simulink model "SOC_EKF"  (R2023b)
settings: Solver=FixedStepAuto  StartTime=0.0  StopTime=3600  RelTol=1e-3
undefined symbols (not defined in the file or in its folder): Ion, Lithium
libraries: autolibrcnetworksystem x4, spsBatteryLib x1, spsSeriesRLCBranchLib x1, spspowerguiLib x1
settings Model: Creator=LEGION  LastModifiedBy=LEGION
settings SolverCC: AlgebraicLoopSolver=TrustRegion
settings DebuggingCC: UnconnectedInputMsg=warning  UnconnectedOutputMsg=warning  UnconnectedLineMsg=warning
settings ModelReferenceCC: EnableRefExpFcnMdlSchedulingChecks=on

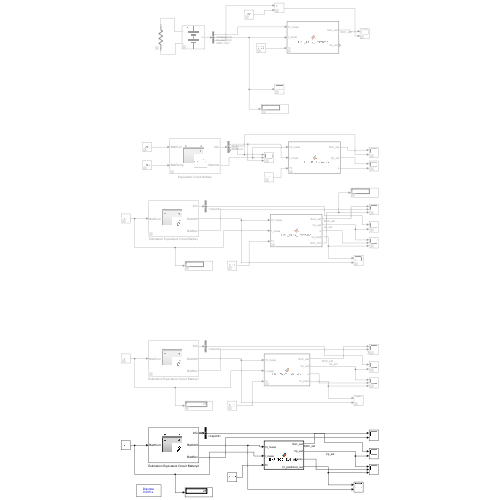
[thumbnail: Simulink's stored preview of the top-level diagram]
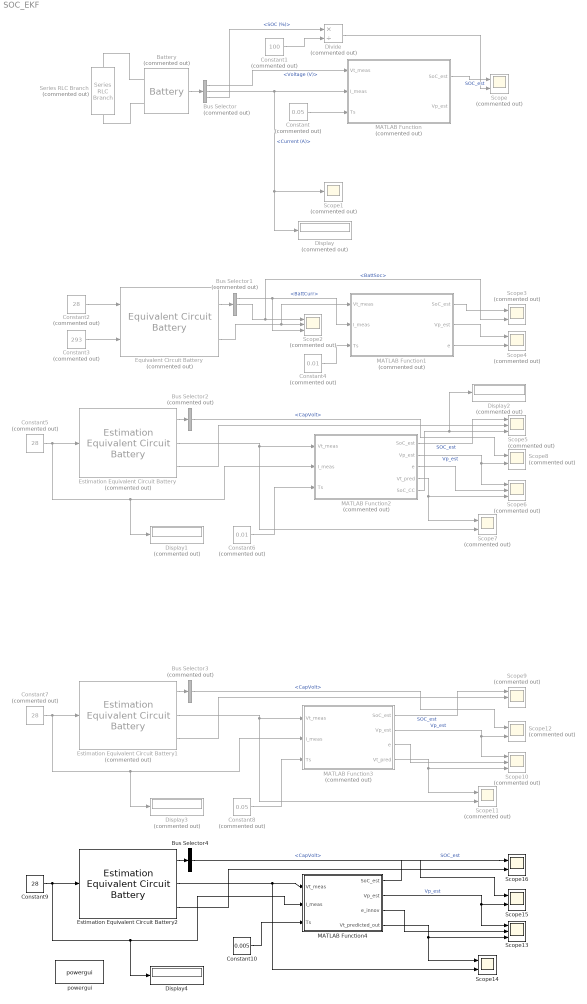
== system SOC_EKF ==
  Battery : spsBatteryLib/Battery  Commented=on  BatType=Lithium-Ion  ShowTempParam=off  ThermalPreset=no  ShowAgeParam=off  NomV=3.7  NomQ=2.3  SOC=85  Batt_Tr=30  PresetModel=on  MaxQ=2.3  MinV=2.775  FullV=4.3068  Dis_rate=1  R=0.016087  Normal_OP=2.08  expZone="[3.9974       0.113]"  current=[6.5 13 32.5]  Units=Time  Tci=20  NomT=20  T2=-30  MaxQ2=4.8  FullV2=7.1  Normal_OP2=5.655  expZone2="[6.58           1]"  Rca=0.6  ti=2000  Dp=0  Neq0=0  Tsim=1e6  Ta1=25  Qeol=5.4*0.9  Reol=0.013333*1.2  Char_age=[2.3478, 3]  Dis_age=[2.3478, 10]  N1=1500  N2=10500  N3=1000  N4=1400  Ta2=45  N5=950
      settings: LibrarySourceBlock=electricdrivelib/Extra Sources/Battery
  Bus Selector : BusSelector  Commented=on  OutputSignals=Voltage (V),Current (A),SOC (%)
  Bus Selector1 : BusSelector  Commented=on  OutputSignals=BattCurr,BattSoc,BattVolt
  Bus Selector2 : BusSelector  Commented=on  OutputSignals=CapVolt
  Bus Selector3 : BusSelector  Commented=on  OutputSignals=CapVolt
  Bus Selector4 : BusSelector  OutputSignals=CapVolt
  Constant : Constant  Commented=on  Value=0.05
  Constant1 : Constant  Commented=on  Value=100
  Constant10 : Constant  Value=0.005
  Constant2 : Constant  Commented=on  Value=28
  Constant3 : Constant  Commented=on  Value=293
  Constant4 : Constant  Commented=on  Value=0.01
  Constant5 : Constant  Commented=on  Value=28
  Constant6 : Constant  Commented=on  Value=0.01
  Constant7 : Constant  Commented=on  Value=28
  Constant8 : Constant  Commented=on  Value=0.05
  Constant9 : Constant  Value=28
  Display{,1..3} (4 alike) : Display  Commented=on
  Display4 : Display
  Divide : Product  Commented=on  Inputs=*/
  Equivalent Circuit Battery : autolibrcnetworksystem/Equivalent Circuit Battery  Commented=on  CapacityCtrl=Parameter  OutputVlt=Unfiltered  NumRC=1  Em=|  R0=|  SOC_BP=|  Temperature_BP=[293.15 313.15]  BattCap=[28 28]  BattCapInit=28  InitialCapVoltage=0  Tc=1/1000  Vinit=4.193  R1=|  C1=|  R2=|  C2=|  R3=|  C3=|  R4=|  C4=|  R5=|  C5=|  Vu=Inf  Vl=-Inf  RefBlkName='autolibrcnetworksystem/Equivalent Circuit Battery'
      Em=|
      | [3.5042 3.5136;
      | 3.5573 3.5646;
      | 3.6009 3.6153;
      | 3.6393 3.6565;
      | 3.6742 3.6889;
      | 3.7121 3.7214;
      | 3.7937 3.8078;
      | 3.8753 3.8945;
      | 3.97 3.9859;
      | 4.0764 4.0821;
      | 4.1924 4.193]
      R0=|
      | [0.011448 0.0090006;
      | 0.011038 0.0089655;
      | 0.011281 0.0091261;
      | 0.011236 0.0091099;
      | 0.010959 0.008957;
      | 0.010714 0.0087969;
      | 0.010698 0.0089126;
      | 0.010712 0.0090517;
      | 0.010917 0.0090444;
      | 0.011304 0.0088992;
      | 0.011603 0.0089015
      | ]
      SOC_BP=|
      | [0
      | 0.1
      | 0.2
      | 0.3
      | 0.4
      | 0.5
      | 0.6
      | 0.7
      | 0.8
      | 0.9
      | 1]
      R1=|
      | [0.010342 0.0012244;
      | 0.0067316 0.0011396;
      | 0.0051156 0.0012661;
      | 0.0043447 0.0012265;
      | 0.0038826 0.0011163;
      | 0.0034226 0.0009968;
      | 0.003346 0.0011458;
      | 0.0033222 0.001345;
      | 0.0033201 0.0013091;
      | 0.0032886 0.0010986;
      | 0.0028114 0.0010309]
      C1=|
      | [2287.7 11897;
      | 6122 24515;
      | 18460 42098;
      | 20975 44453;
      | 15254 33098;
      | 10440 24492;
      | 13903 32975;
      | 16694 40007;
      | 15784 35937;
      | 12165 26430;
      | 9118 24795]
      R2=|
      | [0.010342 0.0012244;
      | 0.0067316 0.0011396;
      | 0.0051156 0.0012661;
      | 0.0043447 0.0012265;
      | 0.0038826 0.0011163;
      | 0.0034226 0.0009968;
      | 0.003346 0.0011458;
      | 0.0033222 0.001345;
      | 0.0033201 0.0013091;
      | 0.0032886 0.0010986;
      | 0.0028114 0.0010309]
      C2=|
      | [2287.7 11897;
      | 6122 24515;
      | 18460 42098;
      | 20975 44453;
      | 15254 33098;
      | 10440 24492;
      | 13903 32975;
      | 16694 40007;
      | 15784 35937;
      | 12165 26430;
      | 9118 24795]
      R3=|
      | [0.010342 0.0012244;
      | 0.0067316 0.0011396;
      | 0.0051156 0.0012661;
      | 0.0043447 0.0012265;
      | 0.0038826 0.0011163;
      | 0.0034226 0.0009968;
      | 0.003346 0.0011458;
      | 0.0033222 0.001345;
      | 0.0033201 0.0013091;
      | 0.0032886 0.0010986;
      | 0.0028114 0.0010309]
      C3=|
      | [2287.7 11897;
      | 6122 24515;
      | 18460 42098;
      | 20975 44453;
      | 15254 33098;
      | 10440 24492;
      | 13903 32975;
      | 16694 40007;
      | 15784 35937;
      | 12165 26430;
      | 9118 24795]
      R4=|
      | [0.010342 0.0012244;
      | 0.0067316 0.0011396;
      | 0.0051156 0.0012661;
      | 0.0043447 0.0012265;
      | 0.0038826 0.0011163;
      | 0.0034226 0.0009968;
      | 0.003346 0.0011458;
      | 0.0033222 0.001345;
      | 0.0033201 0.0013091;
      | 0.0032886 0.0010986;
      | 0.0028114 0.0010309]
      C4=|
      | [2287.7 11897;
      | 6122 24515;
      | 18460 42098;
      | 20975 44453;
      | 15254 33098;
      | 10440 24492;
      | 13903 32975;
      | 16694 40007;
      | 15784 35937;
      | 12165 26430;
      | 9118 24795]
      R5=|
      | [0.010342 0.0012244;
      | 0.0067316 0.0011396;
      | 0.0051156 0.0012661;
      | 0.0043447 0.0012265;
      | 0.0038826 0.0011163;
      | 0.0034226 0.0009968;
      | 0.003346 0.0011458;
      | 0.0033222 0.001345;
      | 0.0033201 0.0013091;
      | 0.0032886 0.0010986;
      | 0.0028114 0.0010309]
      C5=|
      | [2287.7 11897;
      | 6122 24515;
      | 18460 42098;
      | 20975 44453;
      | 15254 33098;
      | 10440 24492;
      | 13903 32975;
      | 16694 40007;
      | 15784 35937;
      | 12165 26430;
      | 9118 24795]
  Estimation Equivalent Circuit Battery : autolibrcnetworksystem/Estimation Equivalent Circuit Battery  Commented=on  NumRC=1  Em=[2.775 3 3.7 3.8 4 4.3068]  R0=[0.01 0.01 0.01 0.01 0.01 0.01]  SOC_BP=[0 .2 .4 .6 .8 1]  BattCap=28  BattCapInit=28  InitialCapVoltage=0  R1=[0.005 0.005 0.005 0.005 0.005 0.005]  C1=[10000 10000 10000 10000 10000 10000]  R2=[0.005 0.005 0.005 0.005 0.005 0.005]  C2=[10000 10000 10000 10000 10000 10000]  R3=[0.005 0.005 0.005 0.005 0.005 0.005]  C3=[10000 10000 10000 10000 10000 10000]  R4=[0.005 0.005 0.005 0.005 0.005 0.005]  C4=[10000 10000 10000 10000 10000 10000]  R5=[0.005 0.005 0.005 0.005 0.005 0.005]  C5=[10000 10000 10000 10000 10000 10000]  Vu=Inf  Vl=-Inf
  Estimation Equivalent Circuit Battery1 : autolibrcnetworksystem/Estimation Equivalent Circuit Battery  Commented=on  NumRC=1  Em=[2.775 3 3.7 3.8 4 4.3068]  R0=[0.01 0.01 0.01 0.01 0.01 0.01]  SOC_BP=[0 .2 .4 .6 .8 1]  BattCap=28  BattCapInit=28  InitialCapVoltage=0  R1=[0.005 0.005 0.005 0.005 0.005 0.005]  C1=[10000 10000 10000 10000 10000 10000]  R2=[0.005 0.005 0.005 0.005 0.005 0.005]  C2=[10000 10000 10000 10000 10000 10000]  R3=[0.005 0.005 0.005 0.005 0.005 0.005]  C3=[10000 10000 10000 10000 10000 10000]  R4=[0.005 0.005 0.005 0.005 0.005 0.005]  C4=[10000 10000 10000 10000 10000 10000]  R5=[0.005 0.005 0.005 0.005 0.005 0.005]  C5=[10000 10000 10000 10000 10000 10000]  Vu=Inf  Vl=-Inf
  Estimation Equivalent Circuit Battery2 : autolibrcnetworksystem/Estimation Equivalent Circuit Battery  NumRC=1  Em=[2.775 3 3.7 3.8 4 4.3068]  R0=[0.01 0.01 0.01 0.01 0.01 0.01]  SOC_BP=[0 .2 .4 .6 .8 1]  BattCap=28  BattCapInit=28  InitialCapVoltage=0  R1=[0.005 0.005 0.005 0.005 0.005 0.005]  C1=[10000 10000 10000 10000 10000 10000]  R2=[0.005 0.005 0.005 0.005 0.005 0.005]  C2=[10000 10000 10000 10000 10000 10000]  R3=[0.005 0.005 0.005 0.005 0.005 0.005]  C3=[10000 10000 10000 10000 10000 10000]  R4=[0.005 0.005 0.005 0.005 0.005 0.005]  C4=[10000 10000 10000 10000 10000 10000]  R5=[0.005 0.005 0.005 0.005 0.005 0.005]  C5=[10000 10000 10000 10000 10000 10000]  Vu=Inf  Vl=-Inf
  MATLAB Function : MATLAB Function  Commented=on  TreatAsAtomicUnit=on
  MATLAB Function1 : MATLAB Function  Commented=on  TreatAsAtomicUnit=on
  MATLAB Function2 : MATLAB Function  Commented=on  TreatAsAtomicUnit=on
  MATLAB Function3 : MATLAB Function  Commented=on  TreatAsAtomicUnit=on
  MATLAB Function4 : MATLAB Function  TreatAsAtomicUnit=on
  Scope{,3..4,7..8,11..12} (7 alike) : Scope  Commented=on  NumInputPorts=2
  Scope1 : Scope  Commented=on
  Scope{2,5..6,9..10} (5 alike) : Scope  Commented=on  NumInputPorts=3
  Scope13 : Scope  NumInputPorts=3
  Scope14 : Scope  NumInputPorts=2
  Scope15 : Scope  NumInputPorts=2
  Scope16 : Scope  NumInputPorts=2
  Series RLC Branch : spsSeriesRLCBranchLib/Series RLC Branch  Commented=on  LConnTagsString=__new0  RConnTagsString=__new0  BranchType=R  Resistance=1  Inductance=1e-3  SetiL0=off  InitialCurrent=0  Capacitance=1e-6  Setx0=off  InitialVoltage=0  Measurements=None
  powergui : spspowerguiLib/powergui  Priority=1  SimulationMode=Discrete  SampleTime=0.005  frequency=60  Iterations=50  frequencyindice=0  Pbase=100e6  ErrMax=1e-4  UnitsV=kV  UnitsW=MW  buscounter=0  FunctionMessages=off  echomessages=off  EnableUseOfTLC=off  CurrentSourceSwitches=off  DisableSnubberDevices=off  DisableRonSwitches=off  DisableVfSwitches=off  DisplayEquations=off  AutomaticDiscreteSolvers=off  SolverType=Tustin/Backward Euler (TBE)  Interpol=off  ExternalGateDelay=off  methode=off  Ts=100  x0status=blocks  SPID=on  SwTol=0  HookPort=off  NonlinearTolerance=1e-4  nMaxIteration=100  ContinueOnMaxIteration=off  RestoreLinks=warning  ResistiveCurrentMeasurement=off  Frange=[0:2:500]  Ylog=off  Xlog=on  ShowGrid=off  save=off  variable=ZData  structure=0  ZoomFFT=off  StartTime=0.0  cycles=1  DisplayStyle=1  fundamental=60  FreqAxis=off  MaxFrequency=1000  frequencyindicesteady=1  RmsSteady=1  display=off
  wires:
  Battery/1 -> Bus Selector/1
  Bus Selector/1 -> MATLAB Function/1(Vt_meas)  "<Voltage (V)>"
  Bus Selector/2 -> Scope1/1, Display/1, MATLAB Function/2(I_meas)  "<Current (A)>"
  Constant/1 -> MATLAB Function/3(Ts)
  MATLAB Function/1(SoC_est) -> Scope/1  "SOC_est"
  Bus Selector/3 -> Divide/1  "<SOC (%)>"
  Divide/1 -> Scope/2
  Constant1/1 -> Divide/2
  Equivalent Circuit Battery/2 -> MATLAB Function1/1(Vt_meas), Scope2/2
  Constant2/1 -> Equivalent Circuit Battery/1
  Constant3/1 -> Equivalent Circuit Battery/2
  Equivalent Circuit Battery/1 -> Bus Selector1/1
  Bus Selector1/2 -> Scope3/2, Scope2/1  "<BattSoc>"
  Bus Selector1/1 -> Scope2/3, MATLAB Function1/2(I_meas)  "<BattCurr>"
  Constant4/1 -> MATLAB Function1/3(Ts)
  MATLAB Function1/1(SoC_est) -> Scope3/1
  MATLAB Function1/2(Vp_est) -> Scope4/1
  MATLAB Function1/3(e) -> Scope4/2
  Estimation Equivalent Circuit Battery/2 -> Scope7/2, MATLAB Function2/1(Vt_meas)
  Constant5/1 -> Display1/1, MATLAB Function2/2(I_meas), Estimation Equivalent Circuit Battery/1
  MATLAB Function2/1(SoC_est) -> Scope5/1  "SOC_est"
  Estimation Equivalent Circuit Battery/3 -> Scope5/2
  MATLAB Function2/2(Vp_est) -> Scope8/2, Scope6/1  "Vp_est"
  MATLAB Function2/3(e) -> Scope6/2
  MATLAB Function2/4(Vt_pred) -> Scope7/1, Scope6/3
  Constant6/1 -> MATLAB Function2/3(Ts)
  MATLAB Function2/5(SoC_CC) -> Display2/1, Scope5/3
  Estimation Equivalent Circuit Battery/1 -> Bus Selector2/1
  Bus Selector2/1 -> Scope8/1  "<CapVolt>"
  Bus Selector3/1 -> Scope12/1  "<CapVolt>"
  MATLAB Function3/4(Vt_pred) -> Scope11/1, Scope10/3
  Estimation Equivalent Circuit Battery1/3 -> Scope9/2
  Constant8/1 -> MATLAB Function3/3(Ts)
  MATLAB Function3/3(e) -> Scope10/2
  MATLAB Function3/2(Vp_est) -> Scope12/2, Scope10/1  "Vp_est"
  Estimation Equivalent Circuit Battery1/1 -> Bus Selector3/1
  Estimation Equivalent Circuit Battery1/2 -> MATLAB Function3/1(Vt_meas), Scope11/2
  MATLAB Function3/1(SoC_est) -> Scope9/1  "SOC_est"
  Constant7/1 -> MATLAB Function3/2(I_meas), Display3/1, Estimation Equivalent Circuit Battery1/1
  Constant9/1 -> MATLAB Function4/2(I_meas), Display4/1, Estimation Equivalent Circuit Battery2/1
  Estimation Equivalent Circuit Battery2/1 -> Bus Selector4/1
  MATLAB Function4/3(e_innov) -> Scope13/2
  MATLAB Function4/1(SoC_est) -> Scope16/1  "SOC_est"
  Estimation Equivalent Circuit Battery2/2 -> Scope14/2, MATLAB Function4/1(Vt_meas)
  MATLAB Function4/2(Vp_est) -> Scope15/2, Scope13/1  "Vp_est"
  MATLAB Function4/4(Vt_predicted_out) -> Scope14/1, Scope13/3
  Estimation Equivalent Circuit Battery2/3 -> Scope16/2
  Bus Selector4/1 -> Scope15/1  "<CapVolt>"
  Constant10/1 -> MATLAB Function4/3(Ts)
  connections:
  Series RLC Branch/LConn1 -- Battery/LConn1
  Series RLC Branch/RConn1 -- Battery/LConn2

== matlab function SOC_EKF/MATLAB Function1 ==
  settings: updateMethod=DISCRETE
  data: Vt_meas input; SoC_est output; I_meas input; Ts input; Vp_est output; e output
function [SoC_est, Vp_est, e] = EKF_SOC_Estimator(Vt_meas, I_meas, Ts)

% ---------------------------- Persistent Variables ----------------------------
persistent x P Q R
persistent SoC_vec Em_chg Em_dis R0_chg R0_dis R1_chg R1_dis C1_table_chg C1_table_dis
persistent BattCapInit initialized

if isempty(initialized)
    initialized = true;

    % 11-point SoC vector (even spacing)
    SoC_vec = linspace(0, 1, 11);

    % Lookup table data
    Em = [3.5042 3.5136;
          3.5573 3.5646;
          3.6009 3.6153;
          3.6393 3.6565;
          3.6742 3.6889;
          3.7121 3.7214;
          3.7937 3.8078;
          3.8753 3.8945;
          3.9700 3.9859;
          4.0764 4.0821;
          4.1924 4.1930];

    R0 = [0.011448 0.0090006;
          0.011038 0.0089655;
          0.011281 0.0091261;
          0.011236 0.0091099;
          0.010959 0.0089570;
          0.010714 0.0087969;
          0.010698 0.0089126;
          0.010712 0.0090517;
          0.010917 0.0090444;
          0.011304 0.0088992;
          0.011603 0.0089015];

    R1 = [0.010342 0.0012244;
          0.0067316 0.0011396;
          0.0051156 0.0012661;
          0.0043447 0.0012265;
          0.0038826 0.0011163;
          0.0034226 0.0009968;
          0.0033460 0.0011458;
          0.0033222 0.0013450;
          0.0033201 0.0013091;
          0.0032886 0.0010986;
          0.0028114 0.0010309];

    C1_table = [2287.7 11897;
                6122   24515;
               18460   42098;
               20975   44453;
               15254   33098;
               10440   24492;
               13903   32975;
               16694   40007;
               15784   35937;
               12165   26430;
                9118   24795];

    % Split into charge/discharge
    Em_dis = Em(:,1); Em_chg = Em(:,2);
    R0_dis = R0(:,1); R0_chg = R0(:,2);
    R1_dis = R1(:,1); R1_chg = R1(:,2);
    C1_table_dis = C1_table(:,1); C1_table_chg = C1_table(:,2);

    % Battery capacity
    BattCapInit = 28;  % [Ah]

    % ---------------- Initial State (Realistic) ----------------
    SoC_init = 1.0;
    Voc_init = Em_dis(end);  % Voc at 100% SoC
    Rt_init  = R0_dis(end);  % Rt at 100% SoC
    Vp_init  = Voc_init - Vt_meas + Rt_init * I_meas;

    x = [SoC_init; Vp_init];

    % Initial covariance
    P = 1e-2 * eye(2);

    % Noise covariance
    Q = diag([1e-4, 1e-3]);
    R = 1e-2;

end

% ---------------------------- Parameter Interpolation ----------------------------
SoC = min(max(x(1), 0), 1);  % Clamp SoC to [0,1]

if I_meas >= 0  % Discharge
    Voc = interp1(SoC_vec, Em_dis, SoC, 'linear', 'extrap');
    Rt  = interp1(SoC_vec, R0_dis, SoC, 'linear', 'extrap');
    Rp  = interp1(SoC_vec, R1_dis, SoC, 'linear', 'extrap');
    Cp  = interp1(SoC_vec, C1_table_dis, SoC, 'linear', 'extrap');
else
    Voc = interp1(SoC_vec, Em_chg, SoC, 'linear', 'extrap');
    Rt  = interp1(SoC_vec, R0_chg, SoC, 'linear', 'extrap');
    Rp  = interp1(SoC_vec, R1_chg, SoC, 'linear', 'extrap');
    Cp  = interp1(SoC_vec, C1_table_chg, SoC, 'linear', 'extrap');
end

Cp = max(Cp, 1e-3);  % Prevent numerical issues

% ---------------------------- Discrete-Time Model ----------------------------
alpha = exp(-Ts / (Rp * Cp));
A = [1, 0;
     0, alpha];
B = [-Ts / (3600 * BattCapInit);
      Rp * (1 - alpha)];

% ---------------------------- EKF PREDICTION ----------------------------
x_pred = A * x + B * I_meas;
P_pred = A * P * A' + Q;

% ---------------------------- Measurement Prediction ----------------------------
Vt_pred = Voc - x_pred(2) + Rt * I_meas;

% ---------------------------- Correction ----------------------------
C_k = [1, -1];
e = Vt_meas - Vt_pred;
S_k = C_k * P_pred * C_k' + R;
K = P_pred * C_k' / S_k;

x = x_pred + K * e;
P = (eye(2) - K * C_k) * P_pred;

% ---------------------------- Output ----------------------------
SoC_est = max(0, min(1, x(1)));
Vp_est  = x(2);
e = Vt_meas - Vt_pred;

end

== matlab function SOC_EKF/MATLAB Function ==
  data: Vt_meas input; SoC_est output; I_meas input; Ts input; Vp_est output
function [SoC_est, Vp_est] = EKF_SOC_Estimator(Vt_meas, I_meas, Ts)

% --- Persistent variables to retain state across time steps ---
persistent x P Q R A B C D Voc0 dVoc C_nom Rp Cp

if isempty(x)
    % Initial state: SoC (0.85) and Vp (0 V)
    x = [0.85; 0];  % [SoC; Vp]

    % Covariance matrix (uncertainty in initial estimate)
    P = 1e-2 * eye(2);

    % Process noise covariance (uncertainty in model)
    Q = diag([1e-6, 1e-4]);

    % Measurement noise covariance (voltage sensor noise)
    R = 1e-3;

    % --- Battery model parameters ---
    C_nom = 2.3;         % Nominal capacity [Ah]
    Rp = 0.01;           % Polarization resistance [Ohm] 
    Cp = 5000;           % Polarization capacitance [F] 
    Rt = 0.016087;       % Ohmic resistance [Ohm] 

    % OCV parameters (linearized)
    Voc0 = 2.775;                      % OCV at SoC = 0
    dVoc = 4.3068 - 2.775;            % Total OCV slope over SoC (≈1.5318 V)

    % --- State-space model (discrete time) ---
    alpha = exp(-Ts / (Rp * Cp));     % Exponential decay of Vp

    A = [1, 0;
         0, alpha];

    B = [-Ts / (3600 * C_nom);
          Rp * (1 - alpha)];

    C = [dVoc, -1];  % Output equation: Vt_est = Voc(SoC) - Vp + I*Rt
    D = Rt;
end

% --- EKF PREDICTION STEP ---
x_pred = A * x + B * I_meas;
P_pred = A * P * A' + Q;

% --- ESTIMATE TERMINAL VOLTAGE ---
Vt_pred = Voc0 + C * x_pred + D * I_meas;

% --- MEASUREMENT UPDATE (INNOVATION) ---
e = Vt_meas - Vt_pred;                    % Innovation (residual)
S = C * P_pred * C' + R;                  % Innovation covariance
K = P_pred * C' / S;                      % Kalman Gain

% --- EKF CORRECTION STEP ---
x = x_pred + K * e;                       % Updated state
P = (eye(2) - K * C) * P_pred;            % Updated covariance

% --- OUTPUT ---
SoC_est = max(0, min(1, x(1)));           % Clamp to [0,1]
Vp_est  = x(2);                           % Estimated Vp

end

== matlab function SOC_EKF/MATLAB Function2 ==
  settings: updateMethod=DISCRETE
  data: Vt_meas input; SoC_est output; I_meas input; Ts input; Vp_est output; e output; Vt_pred output; SoC_CC output
function [SoC_est, Vp_est, e, Vt_pred, SoC_CC] = EKF_SOC_Estimator(Vt_meas, I_meas, Ts)

% --- Persistent variables to retain state across time steps ---
persistent x P Q R C_k SOC_vec Em Rt Rp Cp C_nom initialized SoC_CC_prev

if isempty(initialized)
    initialized = true;

    % Initial SoC
    SOC_init = 1.0;

    % OCV-SOC table (from battery block)
    SOC_vec = [0 0.2 0.4 0.6 0.8 1];
    Em      = [2.775 3 3.7 3.8 4 4.3068];  % Voc [V]

    % Battery constants
    C_nom = 28;       % [Ah]
    Rt = 0.01;        % Series resistance [Ohm]
    Rp = 0.005;       % Polarization resistance [Ohm]
    Cp = 10000;       % Polarization capacitance [F]

    % Initial Voc and Vp estimate
    Voc_init = interp1(SOC_vec, Em, SOC_init, 'linear', 'extrap');
    Vp_init  = Voc_init - Vt_meas + Rt * I_meas;

    % Initial state: [SoC; Vp]
    x = [SOC_init; Vp_init];
    SoC_CC_prev = SOC_init;

    % Kalman Filter matrices
    P = 1e-2 * eye(2);               % Initial covariance
    Q = diag([1e-4, 1e-3]);          % Process noise
    R = 1e-2;                        % Measurement noise
    C_k = [1, -1];                   % Output: Voc - Vp + Rt*I
end

% --- Interpolate Voc from OCV-SOC table ---
SoC = max(0, min(1, x(1)));  % Clamp
Voc = interp1(SOC_vec, Em, SoC, 'linear', 'extrap');

% --- State-space matrices ---
alpha = exp(-Ts / (Rp * Cp));
A = [1, 0;
     0, alpha];
B = [-Ts / (3600 * C_nom);
      Rp * (1 - alpha)];

% --- EKF prediction ---
x_pred = A * x + B * I_meas;
P_pred = A * P * A' + Q;

% --- Terminal voltage prediction ---
Vt_pred = Voc - x_pred(2) + Rt * I_meas;

% --- Innovation ---
e = Vt_meas - Vt_pred;
S_k = C_k * P_pred * C_k' + R;
K = P_pred * C_k' / S_k;

% --- EKF correction ---
x = x_pred + K * e;
P = (eye(2) - K * C_k) * P_pred;

% --- Coulomb Counting Update (with correct sign) ---
% Convention: positive I_meas = discharge → SoC should decrease
delta_SoC = Ts * I_meas / (3600 * C_nom);  % no sign flip needed if I > 0 during discharge
SoC_CC = SoC_CC_prev - delta_SoC;
SoC_CC = max(0, min(1, SoC_CC));  % Clamp
SoC_CC_prev = SoC_CC;

% --- Optional debug output ---
% disp(["I=", I_meas, " delta=", delta_SoC, " SoC_CC=", SoC_CC]);

% --- Final Blended SoC ---
alpha_blend = 0.04;  % Tuning weight
SoC_EKF = max(0, min(1, x(1)));
SoC_est = (1 - alpha_blend) * SoC_EKF + alpha_blend * SoC_CC;

% --- Output ---
Vp_est = x(2);

end

== matlab function SOC_EKF/MATLAB Function3 ==
  settings: updateMethod=DISCRETE  sampleTime=0.05
  data: Vt_meas input; SoC_est output; I_meas input; Ts input; Vp_est output; e output; Vt_pred output
function [SoC_est, Vp_est, e, Vt_pred] = EKF_SOC_Estimator(Vt_meas, I_meas, Ts)

% --- Persistent variables to retain state across time steps ---
persistent x P Q R C_k SOC_vec Em Rt Rp Cp C_nom initialized

if isempty(initialized)
    initialized = true;

    % Initial battery state
    SOC_init = 1.0;

    % OCV-SOC curve from battery model
    SOC_vec = [0 0.2 0.4 0.6 0.8 1];                        % SOC breakpoints
    Em      = [2.775 3 3.7 3.8 4 4.3068];                   % OCV [V]

    % Battery parameters
    C_nom = 28;          % Ah
    Rt = 0.01;           % Series resistance [Ohm]
    Rp = 0.005;          % Polarization resistance [Ohm]
    Cp = 10000;          % Polarization capacitance [F]

    % Initial Voc and Vp
    Voc_init = interp1(SOC_vec, Em, SOC_init, 'linear', 'extrap');
    Vp_init  = Voc_init - Vt_meas + Rt * I_meas;

    % Initial state [SoC; Vp]
    x = [SOC_init; Vp_init];

    % EKF initialization
    P = 1e-2 * eye(2);             % Initial state covariance
    Q = diag([1e-3, 1e-2]);        % Process noise covariance
    R = 1e-2;                      % Measurement noise covariance

    % Output equation: Vt = Voc(SoC) - Vp + I*Rt
    C_k = [1, -1];
end

% --- Interpolate OCV based on current SoC ---
SoC = min(max(x(1), 0), 1);  % Clamp SoC to [0,1]
Voc = interp1(SOC_vec, Em, SoC, 'linear', 'extrap');

% --- Discrete-time system matrices ---
alpha = exp(-Ts / (Rp * Cp));
A = [1, 0;
     0, alpha];
B = [-Ts / (3600 * C_nom);
      Rp * (1 - alpha)];

% --- EKF Prediction ---
x_pred = A * x + B * I_meas;
P_pred = A * P * A' + Q;

% --- Measurement prediction ---
Vt_pred = Voc - x_pred(2) + Rt * I_meas;

% --- Innovation ---
e = Vt_meas - Vt_pred;
S_k = C_k * P_pred * C_k' + R;
K = P_pred * C_k' / S_k;

% --- EKF Correction ---
x = x_pred + K * e;
P = (eye(2) - K * C_k) * P_pred;

% --- Output ---
SoC_est = max(0, min(1, x(1)));  % Clamp to [0,1]
Vp_est  = x(2);                  % Estimated polarization voltage

end

== matlab function SOC_EKF/MATLAB Function4 ==
  settings: updateMethod=DISCRETE  sampleTime=0.05
  data: Vt_meas input; SoC_est output; I_meas input; Ts input; Vp_est output; e_innov output; Vt_predicted_out output
function [SoC_est, Vp_est, e_innov, Vt_predicted_out] = EKF_SOC_Estimator(Vt_meas, I_meas, Ts)
% EKF_SOC_Estimator estimates State of Charge (SOC) and polarization voltage (Vp)
% for a battery using an Extended Kalman Filter.
%
% Inputs:
%   Vt_meas: Measured terminal voltage [V]
%   I_meas:  Measured current [A] (positive for discharge, negative for charge)
%   Ts:      Sample time [s]
%
% Outputs:
%   SoC_est: Estimated State of Charge [0-1]
%   Vp_est:  Estimated polarization voltage [V]
%   e_innov: Innovation (measurement residual) [V]
%   Vt_predicted_out: Predicted terminal voltage [V]

% --- Persistent variables to retain state across time steps ---
persistent x P Q R SOC_lookup Em_lookup Rt_val Rp_val Cp_val C_nominal initialized

if isempty(initialized)
    % --- Battery Parameters ---
    SOC_lookup = [0  0.2  0.4  0.6  0.8  1.0];
    Em_lookup  = [2.775 3.0 3.7 3.8 4.0 4.3068];

    C_nominal = 28.0;
    Rt_val    = 0.01;
    Rp_val    = 0.005;
    Cp_val    = 10000;

    SOC_initial = 1.0;
    Vp_initial  = 0.0;
    x = [SOC_initial; Vp_initial];

    P = diag([1e-4, 1e-3]);
    Q = diag([1e-4, 1e-3]);
    R = 1e-2;

    initialized = true;
end

% 1. State Prediction
alpha = exp(-Ts / (Rp_val * Cp_val));
A = [1,  0;
     0,  alpha];
B = [-Ts / (C_nominal * 3600);
      Rp_val * (1 - alpha)];
x_pred = A * x + B * I_meas;
x_pred(1) = min(max(x_pred(1), 0), 1); % Clamp predicted SoC

% 2. Covariance Prediction
P_pred = A * P * A' + Q;

% 3. Measurement Prediction
SoC_predicted = x_pred(1);
Vp_predicted  = x_pred(2);
Voc_predicted = interp1(SOC_lookup, Em_lookup, SoC_predicted, 'linear', 'extrap');
Vt_predicted = Voc_predicted - Vp_predicted + Rt_val * I_meas;

% 4. Calculate Jacobian of Measurement Function (C_k_val atau H_k)
num_points = length(SOC_lookup);
dVoc_dSoC = 0; % Default fallback slope

if num_points < 2
    % If less than 2 points in lookup table, derivative is undefined or zero
    dVoc_dSoC = 0;
elseif SoC_predicted <= SOC_lookup(1)
    % Extrapolate using the slope of the first segment
    delta_SOC = SOC_lookup(2) - SOC_lookup(1);
    if delta_SOC > 1e-9 % Avoid division by zero
        dVoc_dSoC = (Em_lookup(2) - Em_lookup(1)) / delta_SOC;
    else
        dVoc_dSoC = 0; % Fallback if segment length is zero
    end
elseif SoC_predicted >= SOC_lookup(num_points)
    % Extrapolate using the slope of the last segment
    delta_SOC = SOC_lookup(num_points) - SOC_lookup(num_points-1);
    if delta_SOC > 1e-9
        dVoc_dSoC = (Em_lookup(num_points) - Em_lookup(num_points-1)) / delta_SOC;
    else
        dVoc_dSoC = 0; % Fallback
    end
else
    % SoC_predicted is between SOC_lookup(1) and SOC_lookup(num_points)
    % Find k_loop such that SOC_lookup(k_loop) <= SoC_predicted < SOC_lookup(k_loop+1)
    k_segment = 0; % Initialize index for the segment's start
    for k_loop = 1:(num_points - 1)
        if SoC_predicted >= SOC_lookup(k_loop) && SoC_predicted < SOC_lookup(k_loop+1)
            k_segment = k_loop;
            break;
        end
    end
    
    if k_segment > 0 % A valid segment [k_segment, k_segment+1] is identified
        delta_SOC = SOC_lookup(k_segment+1) - SOC_lookup(k_segment);
        if delta_SOC > 1e-9
            dVoc_dSoC = (Em_lookup(k_segment+1) - Em_lookup(k_segment)) / delta_SOC;
        else
            dVoc_dSoC = 0; % Fallback for zero length segment
        end
    else
        % This part handles the case where SoC_predicted might be exactly SOC_lookup(num_points)
        % which should have been caught by 'SoC_predicted >= SOC_lookup(num_points)'
        % or if no segment was found (should not happen if logic is correct and inputs are valid)
        % As a robust fallback, if SoC_predicted is at the last point, use the last segment's slope.
        if SoC_predicted == SOC_lookup(num_points) && num_points >=2 % num_points >=2 ensures SOC_lookup(num_points-1) is valid
             delta_SOC_last = SOC_lookup(num_points) - SOC_lookup(num_points-1);
             if delta_SOC_last > 1e-9
                dVoc_dSoC = (Em_lookup(num_points) - Em_lookup(num_points-1)) / delta_SOC_last;
             % else dVoc_dSoC remains its current value (likely 0 from initialization)
             end
        % else dVoc_dSoC remains the default (0)
        end
    end
end

% Final check for NaN/Inf (e.g. if delta_SOC was extremely small but not zero)
if isnan(dVoc_dSoC) || isinf(dVoc_dSoC)
    dVoc_dSoC = 0;
end

C_k_val = [dVoc_dSoC, -1];

% 5. Calculate Innovation
e_innov = Vt_meas - Vt_predicted;

% 6. Calculate Innovation Covariance
S_k = C_k_val * P_pred * C_k_val' + R;

% 7. Calculate Kalman Gain
K_k = zeros(2,1); % Initialize K_k
if abs(S_k) > 1e-9 % Check for singularity or very small S_k to avoid division by zero
    K_k = P_pred * C_k_val' / S_k;
end

% 8. State Update
x = x_pred + K_k * e_innov;
x(1) = min(max(x(1), 0), 1); % Clamp corrected SoC

% 9. Covariance Update
P = (eye(2) - K_k * C_k_val) * P_pred;

% --- Output ---
SoC_est = x(1);
Vp_est  = x(2);
Vt_predicted_out = Vt_predicted;

end
